simulink model "et_robocon_zack"  (R2013b)
settings: Solver=ode3  SolverMode=SingleTasking  StartTime=0.0  StopTime=inf  RelTol=1e-3
undefined symbols (not defined in the file): balancerStates_Bus0, current_mode_status, current_task_operation_status, DiscIntNeverNeededParam, Init_Bus0, K, lightCalib, R, STATE, TRACK_MODE_LIST, W
libraries: legonxtlib x19, simulink_extras x4, simulink x3, limbo_algorithm_atomic_sub_chart_library x1, line_tracking_algorithm_atomic_sub_chart_library x1, parking_algorithm_atomic_sub_chart_library x1
(part 2 of 2)

== stateflow chart et_robocon_zack/Main Controller/normal_operation_modes.see_saw_mode ==
  state see_saw_mode
    entry:
    desired_tail = single(1.6);
    BT_status_out = single(0);
    during:
    normalizedLight = processLight(sensors.light,lightCalib);
    PWM.tail = tail_controller(sensors.theta_T, desired_tail);
    state Pause
      entry:
      debugFlag = uint16(601);
    state light = processLight(rawLight,lightCalib) [function]
    state StandUp
      entry: debugFlag = uint16(602);
      initFlags.theta = single(1);
      initFlags.gyroReset = single(1);
      during:
      desired_tail = desired_tail + single(0.0008);
    state Balancing
      state SeesawLogic [parallel]
        settings: executionOrder=1
        state StationnaryBalance
          entry: debugFlag = uint16(603);
          desired_tail = single(0.5);
          initFlags.theta = single(0);
          initFlags.gyroReset = single(0);
          desired_states = balancerStates_Bus0;
        state Approach
          entry: debugFlag = uint16(604);
          during:
          turningPWM = lineTracker(single(-0.3), normalizedLight, single(1.3), sensors.battery);
          exit:
          turningPWM = single(0);
          state StartWalking
            entry:
            entry: debugFlag = uint16(605);
            des_vel = single(0.04);
            during:
            des_vel = des_vel+single(0.00024);
          state Walk
            entry: debugFlag = uint16(605);
          (default) -> StartWalking
          StartWalking -> Walk : [des_vel >= single(0.1)]
        state Seesaw
          entry:
          phi0 = states.phi;
          desired_phi = phi0;
          during:
          turningPWM = phiController(states.phi,desired_phi,sensors.battery);
          exit:
          turningPWM = single(0);
          state turn_around
            entry:
            debugFlag = uint16(606);
            desired_phi = phi0;
            during:
            desired_phi = desired_phi + single(.008);
            turningPWM = phiController(states.phi,desired_phi,sensors.battery);
            exit:
            phi0 = states.phi;
          state JumpOnIt
            entry:
            Speak;
            debugFlag = uint16(606);
            theta_ref = states.balancerStates.theta;
            des_vel = single(0.17);
          state Pause1
          state GoingUP
            entry:
            debugFlag = uint16(607);
            des_vel = single(0.1);
            during:
            turningPWM = phiController(states.phi,desired_phi, sensors.battery)+single(2)*lineTracker(single(0), normalizedLight, single(1), sensors.battery);
            exit:
            des_vel = single(0);
          state WaitForPrincess
            entry:
            entry: debugFlag = uint16(608);
            BT_status_out = single(2);
          state GoingBack
            entry:
            debugFlag = uint16(609);
            des_vel = single(-0.1);
            during:
            exit:
            des_vel = single(0);
          state Pause2
          state WaitForPrincess2
            entry:
            debugFlag = uint16(610);
            BT_status_out = single(3);
          state GoUpAgain
            entry:
            debugFlag = uint16(611);
            des_vel = single(-0.1);
            during:
            exit:
            des_vel = single(0);
          state Pause3
          state Stop
            entry:
            debugFlag = uint16(612);
            BT_status_out = single(4);
          turn_around -> turn_around
          (default) -> JumpOnIt
          JumpOnIt -> GoingUP : [states.balancerStates.theta >= theta_ref+single(2)]
          GoingUP -> Pause1 : [states.balancerStates.theta >= theta_ref + single(17)]
          Pause1 -> WaitForPrincess : after(10,sec)
          WaitForPrincess -> GoingBack : [sensors.BT_status_in == single(102)]
          GoingBack -> Pause2 : [states.balancerStates.theta <= theta_ref + single(6.5)]
          Pause2 -> WaitForPrincess2 : after(10,sec)
          WaitForPrincess2 -> GoUpAgain : [sensors.BT_status_in == single(103)]
          GoUpAgain -> Pause3 : [states.balancerStates.theta <= theta_ref - single(10)]
          Pause3 -> Stop : after(5,sec)
        state RaceDone
          entry: debugFlag = uint16(599);
          current_mode_status = OperationModeStatusEnum.SUCCESSFULLY_COMPLETED;
        (default) -> StationnaryBalance
        StationnaryBalance -> Approach : after(5,sec)
        Approach -> Seesaw : [states.balancerStates.theta_dot<single(-4)  && states.theta_dot_dot < single(-60) ]
      state After [parallel]
        during:
        forwardPWM = balance_ctrl(states.balancerStates, des_vel ,sensors.battery)
        PWM.left = forwardPWM + turningPWM;
        PWM.right = forwardPWM - turningPWM;
        settings: executionOrder=2
    state cmd = phiController(phi,desiredPhi,battery) [function]
    state cmd = lineTracker(desiredLight,light,trackingPower,battery) [function]
    state Speak [function]
    state cmd = tail_controller(current,desired) [function]
    state cmd = balance_ctrl(balancerStates,desired_velocity,battery) [function]
    (default) -> Pause
    Pause -> StandUp : after(3,sec)
    StandUp -> Balancing : [desired_tail >=single(2.0) && sensors.theta_T >= single(2.0)]
  data: rawLight function_input single size=1; lightCalib function_input Bus: Light_Bus size=1; light function_output; cmd function_output; phi function_input single size=1; desiredPhi function_input single size=1; battery function_input double size=1; cmd function_output single size=1; desiredLight function_input single size=1; light function_input single size=1; trackingPower function_input single size=1; battery function_input double size=1; current function_input single size=1; desired function_input single size=1; cmd function_output single size=1; balancerStates function_input Bus: Balancer_States_Bus size=1; desired_velocity function_input single size=1; battery function_input double size=1; cmd function_output single size=1; states input Bus: States_Bus size=1; sensors input Bus: Sensors_Bus size=1; PWM output Bus: PWM_bus size=1; initFlags output Bus: Init_Bus size=1; debugFlag output uint16 size=1; desired_states local Bus: Balancer_States_Bus size=1; desired_tail local single size=1; current_mode_status data_store_memory; balancerStates_Bus0 parameter Bus: Balancer_States_Bus size=1; lightCalib data_store_memory; normalizedLight local single size=1; des_vel local single size=1; theta_ref local single size=1; forwardPWM local single size=1; turningPWM local single size=1; BT_status_out output single size=1; desired_phi local single size=1; phi0 local single size=1

== stateflow chart et_robocon_zack/Main Controller/normal_operation_modes.gyro_calibration_mode ==
  state gyro_calibration_mode
    state wait
      entry:debugFlag = uint16(200);
    state MoveUp
      entry:debugFlag = uint16(201);
      PWM.tail = single(-50);
    state Reset
      entry:debugFlag = uint16(202);
      PWM.tail = single(0);
      initFlags.tail = single(1);
      exit:
      initFlags.tail = single(0);
    state GyroCalibration
      entry:
      desired_tail = single(0);
      during:
      PWM.tail = tail_controller(sensors.theta_T,desired_tail);
      state MoveTailDown
        entry:
        debugFlag = uint16(204);
        during:
        desired_tail = desired_tail + single(0.008);
      state StartCalibration
        entry:
        debugFlag = uint16(205);
        initFlags.gyroInit = single(1);
        initFlags.gyroReset = single(1);
        initFlags.theta = single(1);
      state Wait
        entry: Speak;
      state MakeNoise
        during: Speak;
      state StartCalibration1
        entry:
        debugFlag = uint16(208);
        initFlags.gyroInit = single(0);
        initFlags.gyroReset = single(0);
        initFlags.theta = single(0);
      state CalibComplete
        entry:
        debugFlag = uint16(209);
        current_task_operation_status = OperationModeStatusEnum.SUCCESSFULLY_COMPLETED;
      state cmd = tail_controller(current,desired) [function]
      state Speak [function]
      (default) -> MoveTailDown
      MoveTailDown -> StartCalibration : [desired_tail >= single(1.7)]
      StartCalibration -> Wait : [hasChangedFrom(touch,single(0))]
      Wait -> MakeNoise : after(3,sec)
      MakeNoise -> StartCalibration1 : after(0.5,sec)
      StartCalibration1 -> CalibComplete
    (default) -> wait
    wait -> MoveUp : [hasChangedFrom(touch,single(0))]
    MoveUp -> Reset : after(2,sec)
    Reset -> GyroCalibration : after(1,sec)
  data: current function_input single size=1; desired function_input single size=1; cmd function_output single size=1; debugFlag output uint16 size=1; current_task_operation_status data_store_memory; sensors input Bus: Sensors_Bus size=1; touch input single size=1; initFlags output Bus: Init_Bus size=1; PWM output Bus: PWM_bus size=1; desired_tail local

== stateflow chart et_robocon_zack/Main Controller/normal_operation_modes.light_sensor_calibration_mode ==
  state light_sensor_calibration_mode
    during: PWM.tail = tail_controller(sensors.theta_T,single(1.6))
    state WaitForBlack
      entry: debugFlag = uint16(310);
    state StoreBlack
      entry: lightCalib.black = sensors.light;
      debugFlag = uint16(311);
    state WaitForWhite
      entry: debugFlag = uint16(312)
    state StoreWhite
      entry: lightCalib.white = sensors.light;
      debugFlag = uint16(313);
    state WaitForGo
      entry: debugFlag = uint16(314)
    state CalibComplete
      entry:
      debugFlag = uint16(318);
      current_task_operation_status = OperationModeStatusEnum.SUCCESSFULLY_COMPLETED;
    state cmd = tail_controller(current,desired) [function]
    (default) -> WaitForBlack
    WaitForBlack -> StoreBlack : [hasChangedFrom(touch,single(0))]
    StoreBlack -> WaitForWhite : after(1,sec)
    WaitForWhite -> StoreWhite : [hasChangedFrom(touch,single(0))]
    StoreWhite -> WaitForGo : after(1,sec)
    WaitForGo -> CalibComplete : [hasChangedFrom(touch,single(0))]
  data: current function_input single size=1; desired function_input single size=1; cmd function_output single size=1; sensors input Bus: Sensors_Bus size=1; lightCalib data_store_memory; current_task_operation_status data_store_memory; debugFlag output uint16; touch input single size=1; PWM output Bus: PWM_bus size=1
